simulink model "ysw2_7"  (R2014a)
settings: Solver=ode45  StartTime=0.0  StopTime=10.0  RelTol=1e-3
settings Model: Creator=Administrator  LastModifiedBy=Administrator

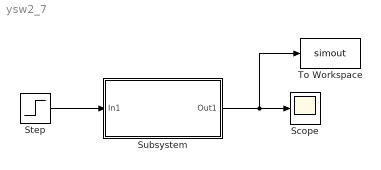
== system ysw2_7 ==
  Scope : Scope
  Step : Step  SampleTime=0
  Subsystem : Subsystem  mask(ysw){zeta=0.707, wn=1}
      mask prompts: zeta "阻尼系数"; wn "无阻尼振荡频率"
      mask help:
      | this is "二阶控制系统"
      | zeta
      | wn
      mask init:
      | zeta=0.707;
      | wn=1;
      mask Help:
      | this is "二阶控制系统"
      | zeta
      | wn
      mask Display:
      | disp('二阶系统')
      | plot([0 1 2 3 10],-exp(-[0 1 2 3 10]))
  To Workspace : ToWorkspace  VariableName=simout  SampleTime=-1
  wires:
  Subsystem/1(Out1) -> To Workspace/1, Scope/1
  Step/1 -> Subsystem/1(In1)

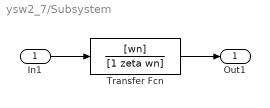
== system ysw2_7/Subsystem ==
  In1 : Inport
  Transfer Fcn : TransferFcn  Numerator=[wn]  Denominator=[1 zeta wn]
  Out1 : Outport
  wires:
  In1/1 -> Transfer Fcn/1
  Transfer Fcn/1 -> Out1/1
